simulink model "Helicopter_MPC"  (R2018a)
settings: Solver=ode4  StartTime=0.0  StopTime=inf  FixedStep=0.1  RelTol=1e-3
values from neighbouring files (symbols this model uses):
  A = [A1;A2;A3;A4]    [Helicopter_Values.m]
  B = [B1;B2;B3;B4]    [Helicopter_Values.m]
  Bp = 0.01    [Helicopter_Values.m]
  By = 0.08    [Helicopter_Values.m]
  g = 9.81    [Helicopter_Values.m]
  jeqp = 0.0172    [Helicopter_Values.m]
  jeqy = 0.021    [Helicopter_Values.m]
  kpp = 0.0556    [Helicopter_Values.m]
  kpy = 0.005    [Helicopter_Values.m]
  kyp = 0.15    [Helicopter_Values.m]
  kyy = 0.21084    [Helicopter_Values.m]
  lcm = 0.015    [Helicopter_Values.m]
  mheli = 0.479    [Helicopter_Values.m]
  p_r_op = -10*pi/180    (= -0.174532925199)    [Helicopter_Values.m]
  Vmp_op = (kyy*mheli*g*cos(p_r_op)*lcm)/(kyy*kpp -kyp*kpy)    [Helicopter_Values.m]
  Vmy_op = kyp*Vmp_op/kyy    [Helicopter_Values.m]
  wp_op = 0    [Helicopter_Values.m]
  wy_op = 0    [Helicopter_Values.m]
  y_r_op = pi/2    (= 1.57079632679)    [Helicopter_Values.m]
undefined symbols (not defined in the file or in its folder): d2r
libraries: mpclib x2, realtime_pacer_lib x1
settings Model: Creator=pacoa  LastModifiedBy=pacoa

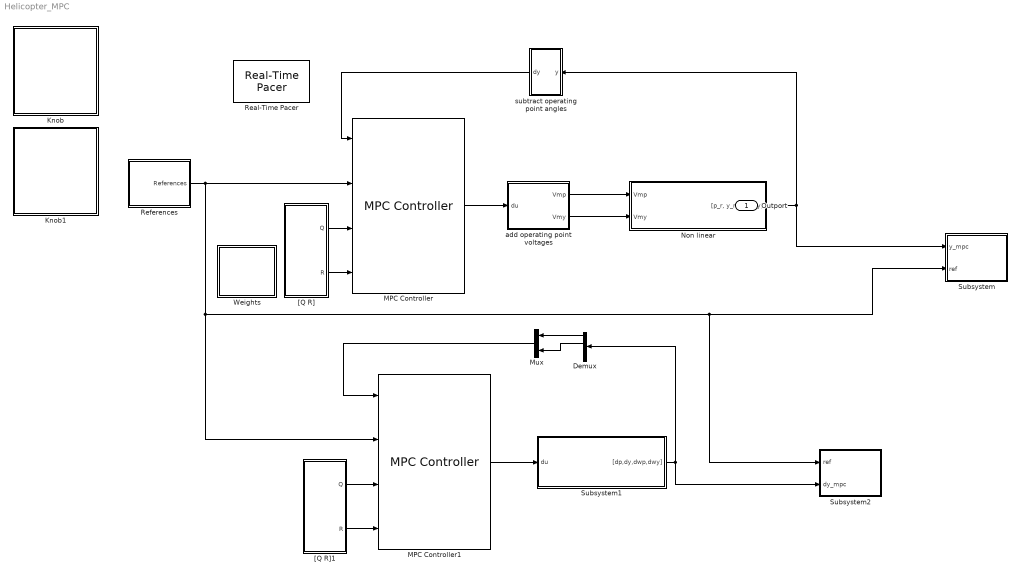
== system Helicopter_MPC ==
  Demux : Demux
  Knob : Subsystem  DialogController=hmiCreateDDGDialog  IsWebBlock=on  mask(MWDashboardBlock){webBlockId=a73d84b2-17ef-427f-b6af-c66f24d9cb1d, webBlockType=continuousknob, ShowInLibBrowser=on, ShowInitialText=on, HMISrcModelName=Helicopter_MPC}
      mask prompts: webBlockId "WebBlock Id"; webBlockType "WebBlock Type"; HMISrcModelName "Source Model"
      mask help: SimulinkHMI:dialogs:ContinuousKnobDialogDesc
      mask Help: helpview([docroot '/mapfiles/simulink.map'], 'hmi_knob')
      mask Display:
      | if strcmp(get_param(bdroot(gcb),'BlockDiagramType'), 'library')
      |     image([(matlabroot) '/toolbox/simulink/hmi/icons/ContinuousKnob.png']);
      | end
  Knob1 : Subsystem  DialogController=hmiCreateDDGDialog  IsWebBlock=on  mask(MWDashboardBlock){webBlockId=13bb11c6-b32b-4dbd-9dce-6f2f36341624, webBlockType=continuousknob, ShowInLibBrowser=on, ShowInitialText=on, HMISrcModelName=Helicopter_MPC}
      mask prompts: webBlockId "WebBlock Id"; webBlockType "WebBlock Type"; HMISrcModelName "Source Model"
      mask help: SimulinkHMI:dialogs:ContinuousKnobDialogDesc
      mask Help: helpview([docroot '/mapfiles/simulink.map'], 'hmi_knob')
      mask Display:
      | if strcmp(get_param(bdroot(gcb),'BlockDiagramType'), 'library')
      |     image([(matlabroot) '/toolbox/simulink/hmi/icons/ContinuousKnob.png']);
      | end
  MPC Controller : mpclib/MPC Controller  SCDEnableBlockLinearizationSpecification=on  mpcobj=mpcobj  is_multiple=0  enable_value=0  return_u0=off  updateMPCinCallerWorkspace=on  ref_from_ws=off  ref_signal_name=[]  ref_preview=off  md_from_ws=off  md_signal_name=[]  md_preview=off  from_project=off  project_file=MPCtask.mat  md_inport=off  mv_inport=off  cost_outport=off  return_sequence=off  return_qpstatus=off  return_state=off  state_inport=off  lims_inport=off  cc_inport=off  ywt_inport=on  is_designfromscratch=0  uwt_inport=on  duwt_inport=off  rhoeps_inport=off  uref_inport=off  n_ts=0.1  n_p=20  n_mv=2  n_md=0  n_ud=0  n_mo=2  n_uo=0  BlockDataType=double  SampleTimeInherited=off  switch_inport=off
  MPC Controller1 : mpclib/MPC Controller  SCDEnableBlockLinearizationSpecification=on  mpcobj=mpcobj  is_multiple=0  enable_value=0  return_u0=off  updateMPCinCallerWorkspace=on  ref_from_ws=off  ref_signal_name=[]  ref_preview=off  md_from_ws=off  md_signal_name=[]  md_preview=off  from_project=off  project_file=MPCtask.mat  md_inport=off  mv_inport=off  cost_outport=off  return_sequence=off  return_qpstatus=off  return_state=off  state_inport=off  lims_inport=off  cc_inport=off  ywt_inport=on  is_designfromscratch=0  uwt_inport=on  duwt_inport=off  rhoeps_inport=off  uref_inport=off  n_ts=0.1  n_p=20  n_mv=2  n_md=0  n_ud=0  n_mo=2  n_uo=0  BlockDataType=double  SampleTimeInherited=off  switch_inport=off
  Mux : Mux  Inputs=2
  Non linear : Subsystem
  Real-Time Pacer : realtime_pacer_lib/Real-Time Pacer  simTimePerRealTime=10
  References : Subsystem
  Subsystem : Subsystem
  Subsystem1 : Subsystem
  Subsystem2 : Subsystem
  Weights : Subsystem
  "[Q R]" : Subsystem
  "[Q R]1" : Subsystem
  add operating point voltages : Subsystem
  subtract operating point angles : Subsystem
  Outport : Outport
  wires:
  Non linear/1("[p_r, y_r ,wp, wy]") -> Subsystem/1(y_mpc), subtract operating point angles/1("y ")
  "[Q R]"/1(Q) -> MPC Controller/3
  "[Q R]"/2(R) -> MPC Controller/4
  References/1(References) -> Subsystem2/1(ref), Subsystem/2(ref), MPC Controller1/2, MPC Controller/2
  MPC Controller/1 -> add operating point voltages/1("du ")
  add operating point voltages/1(Vmp) -> Non linear/1(Vmp)
  add operating point voltages/2(Vmy) -> Non linear/2(Vmy)
  subtract operating point angles/1(dy) -> MPC Controller/1
  "[Q R]1"/1(Q) -> MPC Controller1/3
  "[Q R]1"/2(R) -> MPC Controller1/4
  Subsystem1/1("[dp,dy,dwp,dwy]") -> Demux/1, Subsystem2/2(dy_mpc)
  MPC Controller1/1 -> Subsystem1/1(du)
  Demux/1 -> Mux/1
  Demux/2 -> Mux/2
  Mux/1 -> MPC Controller1/1

== system Helicopter_MPC/Knob ==

== system Helicopter_MPC/Knob1 ==

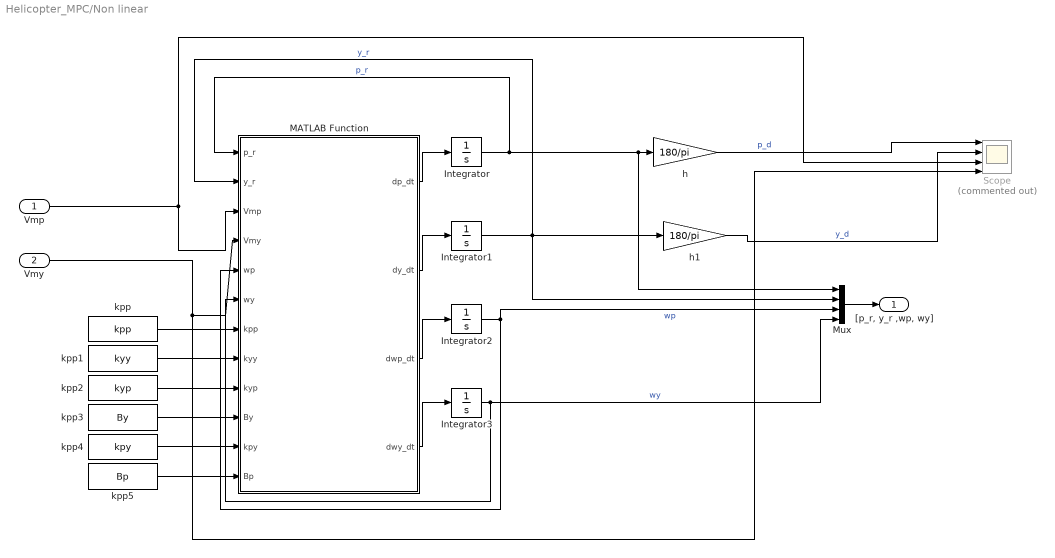
== system Helicopter_MPC/Non linear ==
  Vmp : Inport
  Vmy : Inport  Port=2
  Integrator : Integrator  InitialCondition=d2r(-31.0537918783631)  LimitOutput=on  UpperSaturationLimit=pi/4  LowerSaturationLimit=-pi/4
  Integrator1 : Integrator  InitialCondition=d2r(120.519928781055)  LimitOutput=on  UpperSaturationLimit=pi  LowerSaturationLimit=0
  Integrator2 : Integrator  UpperSaturationLimit=1  LowerSaturationLimit=-1
  Integrator3 : Integrator
  MATLAB Function : MATLAB Function  TreatAsAtomicUnit=on
  Mux : Mux
  Scope : Scope  Commented=on  NumInputPorts=4
  h : Gain  Gain=180/pi
  h1 : Gain  Gain=180/pi
  kpp : Constant  Value=kpp
  kpp1 : Constant  Value=kyy
  kpp2 : Constant  Value=kyp
  kpp3 : Constant  Value=By
  kpp4 : Constant  Value=kpy
  kpp5 : Constant  Value=Bp
  "[p_r, y_r ,wp, wy]" : Outport
  wires:
  Vmy/1 -> Scope/4, MATLAB Function/4(Vmy)
  MATLAB Function/2(dy_dt) -> Integrator1/1
  kpp1/1 -> MATLAB Function/8(kyy)
  Vmp/1 -> MATLAB Function/3(Vmp), Scope/3
  MATLAB Function/4(dwy_dt) -> Integrator3/1
  h1/1 -> Scope/2  "y_d"
  Integrator2/1 -> Mux/3, MATLAB Function/5(wp)  "wp"
  MATLAB Function/3(dwp_dt) -> Integrator2/1
  Integrator1/1 -> h1/1, Mux/2, MATLAB Function/2(y_r)  "y_r"
  h/1 -> Scope/1  "p_d"
  Integrator/1 -> Mux/1, h/1, MATLAB Function/1(p_r)  "p_r"
  kpp4/1 -> MATLAB Function/11(kpy)
  kpp2/1 -> MATLAB Function/9(kyp)
  kpp/1 -> MATLAB Function/7(kpp)
  MATLAB Function/1(dp_dt) -> Integrator/1
  Integrator3/1 -> Mux/4, MATLAB Function/6(wy)  "wy"
  kpp5/1 -> MATLAB Function/12(Bp)
  kpp3/1 -> MATLAB Function/10(By)
  Mux/1 -> "[p_r, y_r ,wp, wy]"/1

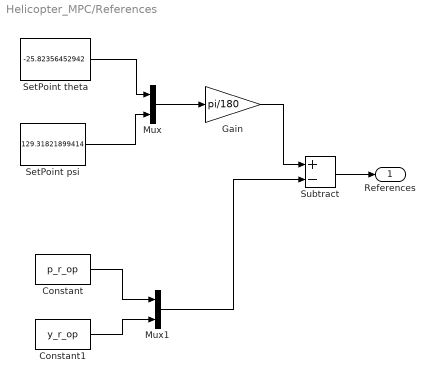
== system Helicopter_MPC/References ==
  Constant : Constant  Value=p_r_op
  Constant1 : Constant  Value=y_r_op
  Gain : Gain  Gain=pi/180
  Mux : Mux  Inputs=2
  Mux1 : Mux  Inputs=2
  SetPoint psi : Constant  Value=129.31821899414
  SetPoint theta : Constant  Value=-25.82356452942
  Subtract : Sum  Inputs=+-
  References : Outport
  wires:
  SetPoint theta/1 -> Mux/1
  SetPoint psi/1 -> Mux/2
  Constant/1 -> Mux1/1
  Constant1/1 -> Mux1/2
  Mux/1 -> Gain/1
  Gain/1 -> Subtract/1
  Mux1/1 -> Subtract/2
  Subtract/1 -> References/1

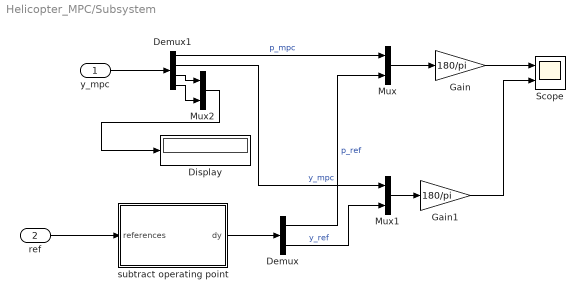
== system Helicopter_MPC/Subsystem ==
  y_mpc : Inport
  ref : Inport  Port=2
  Demux : Demux  Outputs=2
  Demux1 : Demux
  Display : Display
  Gain : Gain  Gain=180/pi
  Gain1 : Gain  Gain=180/pi
  Mux : Mux  Inputs=2
  Mux1 : Mux  Inputs=2
  Mux2 : Mux  Inputs=2
  Scope : Scope  NumInputPorts=2
  "subtract operating point " : Subsystem
  wires:
  Gain1/1 -> Scope/2
  Mux/1 -> Gain/1
  "subtract operating point "/1(dy) -> Demux/1
  Mux1/1 -> Gain1/1
  Demux1/2 -> Mux1/1  "y_mpc"
  Demux/2 -> Mux1/2  "y_ref"
  Gain/1 -> Scope/1
  Demux/1 -> Mux/2  "p_ref"
  Demux1/1 -> Mux/1  "p_mpc"
  y_mpc/1 -> Demux1/1
  ref/1 -> "subtract operating point "/1("references ")
  Demux1/3 -> Mux2/1
  Demux1/4 -> Mux2/2
  Mux2/1 -> Display/1

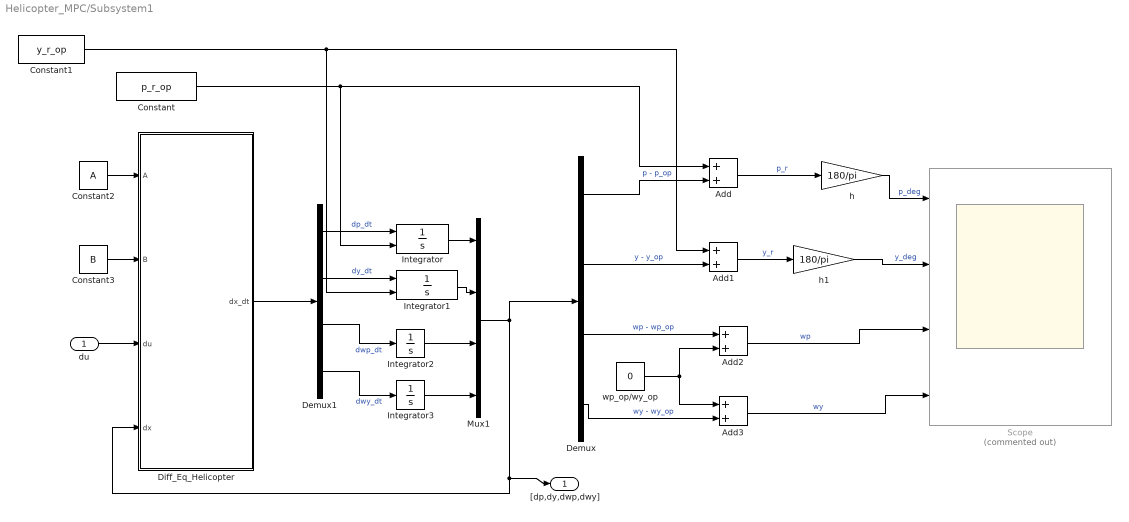
== system Helicopter_MPC/Subsystem1 ==
  du : Inport
  Add{,1..3} (4 alike) : Sum
  Constant : Constant  Value=p_r_op
  Constant1 : Constant  Value=y_r_op
  Constant2 : Constant  Value=A
  Constant3 : Constant  Value=B
  Demux : Demux
  Demux1 : Demux
  Diff_Eq_Helicopter : MATLAB Function  TreatAsAtomicUnit=on
  Integrator : Integrator  InitialConditionSource=external  InitialCondition=-10*pi/180  LimitOutput=on  UpperSaturationLimit=pi/4 - (-10*pi/180)  LowerSaturationLimit=-pi/4 - (-10*pi/180)
  Integrator1 : Integrator  InitialConditionSource=external  InitialCondition=pi/2  LimitOutput=on  UpperSaturationLimit=pi - (pi/2)  LowerSaturationLimit=0 - (pi/2)
  Integrator2 : Integrator  UpperSaturationLimit=pi
  Integrator3 : Integrator
  Mux1 : Mux
  Scope : Scope  Commented=on  NumInputPorts=4
  h : Gain  Gain=180/pi
  h1 : Gain  Gain=180/pi
  wp_op/wy_op : Constant  Value=0
  "[dp,dy,dwp,dwy]" : Outport
  wires:
  Add/1 -> h/1  "p_r"
  Diff_Eq_Helicopter/1(dx_dt) -> Demux1/1
  Constant1/1 -> Integrator1/2, Add1/1
  Integrator1/1 -> Mux1/2
  du/1 -> Diff_Eq_Helicopter/3(du)
  Demux/3 -> Add2/1  "wp - wp_op"
  Demux1/1 -> Integrator/1  "dp_dt"
  Demux1/4 -> Integrator3/1  "dwy_dt"
  Demux/4 -> Add3/2  "wy - wy_op"
  h1/1 -> Scope/2  "y_deg"
  Integrator2/1 -> Mux1/3
  h/1 -> Scope/1  "p_deg"
  Add2/1 -> Scope/3  "wp"
  Demux/1 -> Add/2  "p - p_op"
  Add1/1 -> h1/1  "y_r"
  Demux1/3 -> Integrator2/1  "dwp_dt"
  Constant/1 -> Integrator/2, Add/1
  Demux/2 -> Add1/2  "y - y_op"
  Integrator/1 -> Mux1/1
  Mux1/1 -> Demux/1, "[dp,dy,dwp,dwy]"/1, Diff_Eq_Helicopter/4(dx)
  Demux1/2 -> Integrator1/1  "dy_dt"
  Integrator3/1 -> Mux1/4
  Add3/1 -> Scope/4  "wy"
  wp_op/wy_op/1 -> Add2/2, Add3/1
  Constant2/1 -> Diff_Eq_Helicopter/1(A)
  Constant3/1 -> Diff_Eq_Helicopter/2(B)

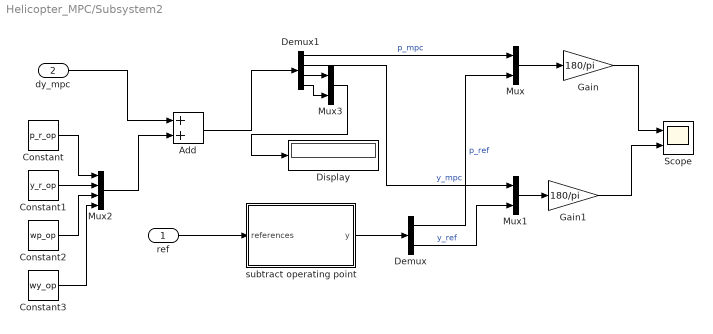
== system Helicopter_MPC/Subsystem2 ==
  ref : Inport
  dy_mpc : Inport  Port=2
  Add : Sum
  Constant : Constant  Value=p_r_op
  Constant1 : Constant  Value=y_r_op
  Constant2 : Constant  Value=wp_op
  Constant3 : Constant  Value=wy_op
  Demux : Demux  Outputs=2
  Demux1 : Demux
  Display : Display
  Gain : Gain  Gain=180/pi
  Gain1 : Gain  Gain=180/pi
  Mux : Mux  Inputs=2
  Mux1 : Mux  Inputs=2
  Mux2 : Mux
  Mux3 : Mux  Inputs=2
  Scope : Scope  NumInputPorts=2
  "subtract operating point " : Subsystem
  wires:
  Gain1/1 -> Scope/2
  Mux/1 -> Gain/1
  "subtract operating point "/1(y) -> Demux/1
  Mux1/1 -> Gain1/1
  Demux1/2 -> Mux1/1  "y_mpc"
  Demux/2 -> Mux1/2  "y_ref"
  Gain/1 -> Scope/1
  Demux/1 -> Mux/2  "p_ref"
  Demux1/1 -> Mux/1  "p_mpc"
  dy_mpc/1 -> Add/1
  ref/1 -> "subtract operating point "/1("references ")
  Constant/1 -> Mux2/1
  Constant1/1 -> Mux2/2
  Constant2/1 -> Mux2/3
  Constant3/1 -> Mux2/4
  Mux2/1 -> Add/2
  Add/1 -> Demux1/1
  Demux1/3 -> Mux3/1
  Demux1/4 -> Mux3/2
  Mux3/1 -> Display/1

== system Helicopter_MPC/Weights ==
  Slider : Subsystem  DialogController=hmiCreateDDGDialog  IsWebBlock=on  mask(MWDashboardBlock){webBlockId=cd9ce9e6-d897-49bc-9bd0-4bcdc8803255, webBlockType=slider, ShowInLibBrowser=on, ShowInitialText=on, HMISrcModelName=Helicopter_MPC}
      mask prompts: webBlockId "WebBlock Id"; webBlockType "WebBlock Type"; HMISrcModelName "Source Model"
      mask help: SimulinkHMI:dialogs:SliderDialogDesc
      mask Help: helpview([docroot '/mapfiles/simulink.map'], 'hmi_slider')
      mask Display:
      | if strcmp(get_param(bdroot(gcb),'BlockDiagramType'), 'library')
      |     image([(matlabroot) '/toolbox/simulink/hmi/icons/Slider.png']);
      | end
  Slider1 : Subsystem  DialogController=hmiCreateDDGDialog  IsWebBlock=on  mask(MWDashboardBlock){webBlockId=fe4bf275-64e4-4d77-b08e-b231e1b5a371, webBlockType=slider, ShowInLibBrowser=on, ShowInitialText=on, HMISrcModelName=Helicopter_MPC}
      mask prompts: webBlockId "WebBlock Id"; webBlockType "WebBlock Type"; HMISrcModelName "Source Model"
      mask help: SimulinkHMI:dialogs:SliderDialogDesc
      mask Help: helpview([docroot '/mapfiles/simulink.map'], 'hmi_slider')
      mask Display:
      | if strcmp(get_param(bdroot(gcb),'BlockDiagramType'), 'library')
      |     image([(matlabroot) '/toolbox/simulink/hmi/icons/Slider.png']);
      | end
  Slider2 : Subsystem  DialogController=hmiCreateDDGDialog  IsWebBlock=on  mask(MWDashboardBlock){webBlockId=c0f9e069-8fb9-4712-95b9-1c600585db0a, webBlockType=slider, ShowInLibBrowser=on, ShowInitialText=on, HMISrcModelName=Helicopter_MPC}
      mask prompts: webBlockId "WebBlock Id"; webBlockType "WebBlock Type"; HMISrcModelName "Source Model"
      mask help: SimulinkHMI:dialogs:SliderDialogDesc
      mask Help: helpview([docroot '/mapfiles/simulink.map'], 'hmi_slider')
      mask Display:
      | if strcmp(get_param(bdroot(gcb),'BlockDiagramType'), 'library')
      |     image([(matlabroot) '/toolbox/simulink/hmi/icons/Slider.png']);
      | end
  Slider3 : Subsystem  DialogController=hmiCreateDDGDialog  IsWebBlock=on  mask(MWDashboardBlock){webBlockId=1237951a-69a5-487f-9f6b-6c59c7967e88, webBlockType=slider, ShowInLibBrowser=on, ShowInitialText=on, HMISrcModelName=Helicopter_MPC}
      mask prompts: webBlockId "WebBlock Id"; webBlockType "WebBlock Type"; HMISrcModelName "Source Model"
      mask help: SimulinkHMI:dialogs:SliderDialogDesc
      mask Help: helpview([docroot '/mapfiles/simulink.map'], 'hmi_slider')
      mask Display:
      | if strcmp(get_param(bdroot(gcb),'BlockDiagramType'), 'library')
      |     image([(matlabroot) '/toolbox/simulink/hmi/icons/Slider.png']);
      | end

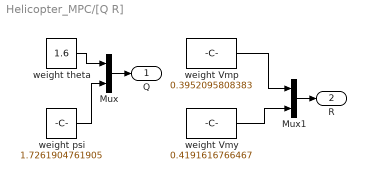
== system Helicopter_MPC/[Q R] ==
  Mux : Mux  Inputs=2
  Mux1 : Mux  Inputs=2
  weight Vmp : Constant  Value=0.3952095808383
  weight Vmy : Constant  Value=0.4191616766467
  weight psi : Constant  Value=1.7261904761905
  weight theta : Constant  Value=1.6
  Q : Outport
  R : Outport  Port=2
  wires:
  weight Vmy/1 -> Mux1/2
  weight psi/1 -> Mux/2
  weight theta/1 -> Mux/1
  weight Vmp/1 -> Mux1/1
  Mux1/1 -> R/1
  Mux/1 -> Q/1

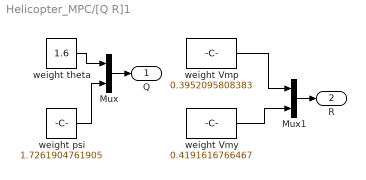
== system Helicopter_MPC/[Q R]1 ==
  Mux : Mux  Inputs=2
  Mux1 : Mux  Inputs=2
  weight Vmp : Constant  Value=0.3952095808383
  weight Vmy : Constant  Value=0.4191616766467
  weight psi : Constant  Value=1.7261904761905
  weight theta : Constant  Value=1.6
  Q : Outport
  R : Outport  Port=2
  wires:
  weight Vmy/1 -> Mux1/2
  weight psi/1 -> Mux/2
  weight theta/1 -> Mux/1
  weight Vmp/1 -> Mux1/1
  Mux1/1 -> R/1
  Mux/1 -> Q/1

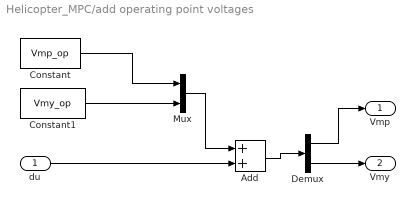
== system Helicopter_MPC/add operating point voltages ==
  "du " : Inport
  Add : Sum
  Constant : Constant  Value=Vmp_op
  Constant1 : Constant  Value=Vmy_op
  Demux : Demux  Outputs=2
  Mux : Mux  Inputs=2
  Vmp : Outport
  Vmy : Outport  Port=2
  wires:
  Constant/1 -> Mux/1
  Constant1/1 -> Mux/2
  Mux/1 -> Add/1
  "du "/1 -> Add/2
  Add/1 -> Demux/1
  Demux/1 -> Vmp/1
  Demux/2 -> Vmy/1

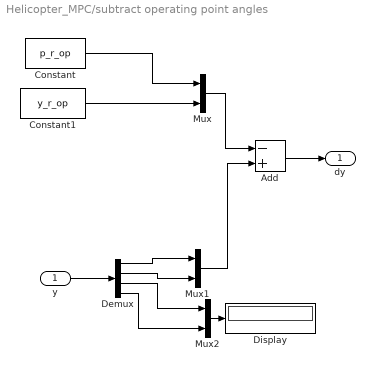
== system Helicopter_MPC/subtract operating point angles ==
  "y " : Inport
  Add : Sum  Inputs=-+
  Constant : Constant  Value=p_r_op
  Constant1 : Constant  Value=y_r_op
  Demux : Demux
  Display : Display
  Mux : Mux  Inputs=2
  Mux1 : Mux  Inputs=2
  Mux2 : Mux  Inputs=2
  dy : Outport
  wires:
  Constant/1 -> Mux/1
  Constant1/1 -> Mux/2
  Mux/1 -> Add/1
  Add/1 -> dy/1
  "y "/1 -> Demux/1
  Demux/1 -> Mux1/1
  Demux/2 -> Mux1/2
  Mux1/1 -> Add/2
  Demux/3 -> Mux2/1
  Demux/4 -> Mux2/2
  Mux2/1 -> Display/1

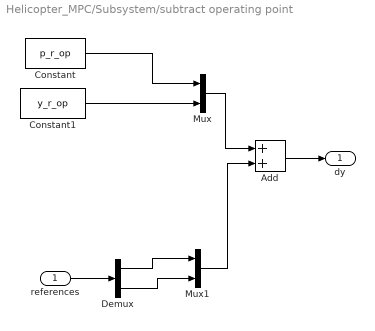
== system Helicopter_MPC/Subsystem/subtract operating point  ==
  "references " : Inport
  Add : Sum
  Constant : Constant  Value=p_r_op
  Constant1 : Constant  Value=y_r_op
  Demux : Demux  Outputs=2
  Mux : Mux  Inputs=2
  Mux1 : Mux  Inputs=2
  dy : Outport
  wires:
  Constant/1 -> Mux/1
  Constant1/1 -> Mux/2
  Mux/1 -> Add/1
  Add/1 -> dy/1
  "references "/1 -> Demux/1
  Demux/1 -> Mux1/1
  Demux/2 -> Mux1/2
  Mux1/1 -> Add/2

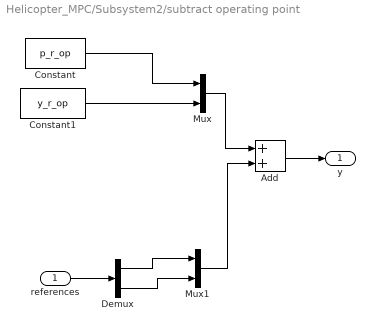
== system Helicopter_MPC/Subsystem2/subtract operating point  ==
  "references " : Inport
  Add : Sum
  Constant : Constant  Value=p_r_op
  Constant1 : Constant  Value=y_r_op
  Demux : Demux  Outputs=2
  Mux : Mux  Inputs=2
  Mux1 : Mux  Inputs=2
  y : Outport
  wires:
  Constant/1 -> Mux/1
  Constant1/1 -> Mux/2
  Mux/1 -> Add/1
  Add/1 -> y/1
  "references "/1 -> Demux/1
  Demux/1 -> Mux1/1
  Demux/2 -> Mux1/2
  Mux1/1 -> Add/2

== system Helicopter_MPC/Weights/Slider ==

== system Helicopter_MPC/Weights/Slider1 ==

== system Helicopter_MPC/Weights/Slider2 ==

== system Helicopter_MPC/Weights/Slider3 ==

== matlab function Helicopter_MPC/Non linear/MATLAB Function ==
  data: p_r input; y_r input; Vmp input; Vmy input; wp input; dp_dt output size=[1 1]; wy input; dy_dt output size=[1 1]; dwp_dt output size=[1 1]; dwy_dt output size=[1 1]; lcm parameter; mheli parameter; jeqp parameter; jeqy parameter; g parameter; kpp input; kyy input; kyp input; By input; kpy input; Bp input
function [dp_dt, dy_dt, dwp_dt, dwy_dt]= fcn(p_r,y_r,Vmp, Vmy,wp,wy, lcm, mheli, jeqp, jeqy, g, kpp, kyy, kyp, By, kpy, Bp)

  %%Parameters
%   
%   Bp,
%   By,
%   g,
%   kpp,
%   kyp,
%   kyy,
%   kpy,
%   mheli,
%   lcm,
%   jeqp,
%   jeqy,
  

%%
   dp_dt = wp;
   dy_dt = wy;
   
   %%
   dwp_dt_n1 = (kpp*Vmp);
   dwp_dt_n2 = (kpy*Vmy);
   dwp_dt_n3 = (Bp*wp+ (mheli*(wy.^2)*sin(p_r)*(lcm^2)*cos(p_r) + (mheli*g*cos(p_r)*lcm)));
   
   dwp_dt_d = (jeqp + mheli*(lcm^2));
   
   dwp_dt = (dwp_dt_n1 -dwp_dt_n2 - dwp_dt_n3)/(dwp_dt_d);
   
   %%
   dwy_dt_n1 = kyp*Vmp;
   dwy_dt_n2 = kyy*Vmy;
   dwy_dt_n3 = 2*mheli*(wy)*sin(p_r)*(lcm^2)*cos(p_r)*wp;
   dwy_dt_n4 = By*wy;
   
   dwy_dt_d = jeqy + mheli*((cos(p_r))^2)*(lcm^2);
   
   dwy_dt = (dwy_dt_n1 - dwy_dt_n2 + dwy_dt_n3 -dwy_dt_n4)/(dwy_dt_d);

== matlab function Helicopter_MPC/Subsystem1/Diff_Eq_Helicopter ==
  data: A input; B input; du input size=[2 1]; dx_dt output; dx input size=[4 1]
function dx_dt = fcn(A,B,du,dx)

dx_dt =A*dx + B*(du);
